simulink model "PIDcontrol"  (Simulink 8.9)
settings: Solver=ode3  StartTime=0.0  StopTime=inf  FixedStep=0.001  RelTol=1e-3  EnableMultiTasking=on
libraries: slrtlib x4, xpcquanserlib x2
settings Model: Creator=Ninad  LastModifiedBy=Rorro  SimulationMode=external
settings SolverCC: EnableConcurrentExecution=on
settings OptimizationCC: BlockReduction=off  OptimizeBlockIOStorage=off  BufferReuse=off  GlobalBufferReuse=off  ExpressionFolding=off  ExpressionDepthLimit=2147483647  LocalBlockOutputs=off
settings DebuggingCC: SolverPrmCheckMsg=warning
settings HardwareCC: ProdIntDivRoundTo=Zero  ProdEndianess=LittleEndian  ProdLongLongMode=on  ProdHWDeviceType=Generic->32-bit x86 compatible
settings RTWCC: SystemTargetFile=slrt.tlc  TemplateMakefile=slrt_default_tmf  Description=Simulink Real-Time  CodeExecutionProfiling=on  RTWCompilerOptimization=on
settings SimulinkRealTimeCC: GeneratePreprocessorConditionals=Disable all
settings ConfigComp: CovSFcnEnable=off

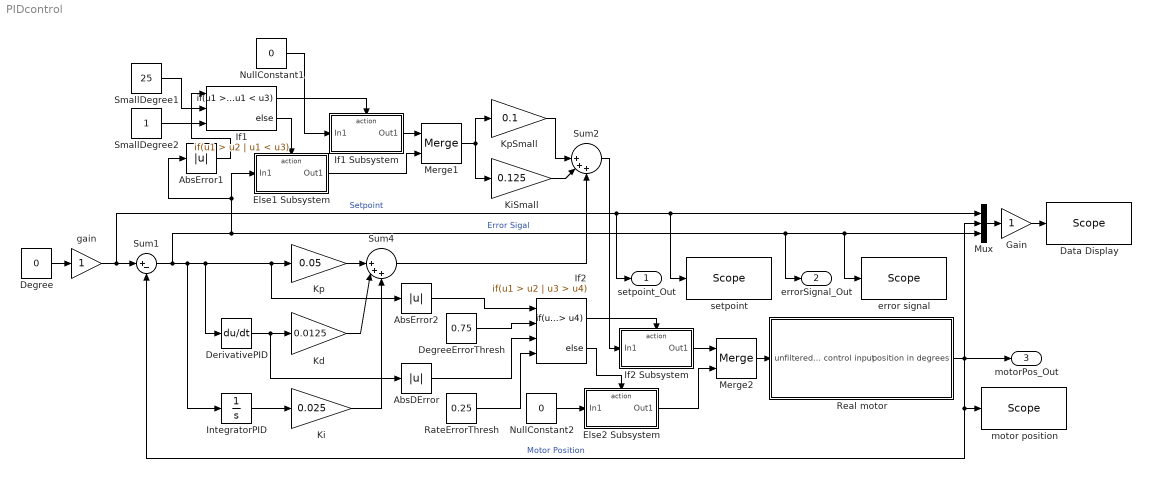
== system PIDcontrol ==
  AbsDError : Abs
  AbsError1 : Abs
  AbsError2 : Abs
  Data Display : slrtlib/Displays and Logging/Scope   scopeno=3  scopetype=Target  autostart=on  viewmode=Numerical  formatstr="'Setpoint        %3.2f,Motor Position  %3.2f,Error Signal    %3.2f'"  grid=on  ylimits=[0,170]  nosamples=200  noprepostsamples=0  interleave=10  triggermode=FreeRun  triggersignal=1  trigsignalfromport=off  triggerlevel=0.0  triggerslope=Either  triggerscope=1  triggersample=0  filename=data.dat  mode=Lazy  writesize=512  autorestart=off  dynamicfilemode=off  maxwritefilesize=512*1024^2
  Degree : Constant  Value=0
  DegreeErrorThresh : Constant  Value=0.75
  DerivativePID : Derivative
  Else1 Subsystem : Subsystem  TreatAsAtomicUnit=on
  Else2 Subsystem : Subsystem  TreatAsAtomicUnit=on
  Gain : Gain
  If1 : If  NumInputs=3  IfExpression=u1 > u2 | u1 < u3
  If1 Subsystem : Subsystem  TreatAsAtomicUnit=on
  If2 : If  NumInputs=4  IfExpression=u1 > u2 | u3 > u4
  If2 Subsystem : Subsystem  TreatAsAtomicUnit=on
  IntegratorPID : Integrator
  Kd : Gain  Gain=0.0125
  Ki : Gain  Gain=0.025
  KiSmall : Gain  Gain=0.125
  Kp : Gain  Gain=0.05
  KpSmall : Gain  Gain=0.1
  Merge1 : Merge
  Merge2 : Merge
  Mux : Mux  Inputs=3
  NullConstant1 : Constant  Value=0
  NullConstant2 : Constant  Value=0
  RateErrorThresh : Constant  Value=0.25
  Real motor : Subsystem
  SmallDegree1 : Constant  Value=25
  SmallDegree2 : Constant
  Sum1 : Sum  Inputs=|+-
  Sum2 : Sum  Inputs=||+++
  Sum4 : Sum  Inputs=||+++
  error signal : slrtlib/Displays and Logging/Scope   scopeno=2  scopetype=Target  autostart=on  viewmode=Graphical rolling  formatstr='%15.6f'  grid=on  ylimits=[-180,180]  nosamples=500  noprepostsamples=0  interleave=10  triggermode=FreeRun  triggersignal=1  trigsignalfromport=off  triggerlevel=0.0  triggerslope=Either  triggerscope=1  triggersample=0  filename=data.dat  mode=Lazy  writesize=512  autorestart=off  dynamicfilemode=off  maxwritefilesize=512*1024^2
  gain : Gain
  motor position : slrtlib/Displays and Logging/Scope   scopeno=7  scopetype=Target  autostart=on  viewmode=Graphical rolling  formatstr='%15.6f'  grid=on  ylimits=[-180,180]  nosamples=500  noprepostsamples=0  interleave=10  triggermode=FreeRun  triggersignal=1  trigsignalfromport=off  triggerlevel=0.0  triggerslope=Either  triggerscope=1  triggersample=0  filename=data.dat  mode=Lazy  writesize=512  autorestart=off  dynamicfilemode=off  maxwritefilesize=512*1024^2
  setpoint : slrtlib/Displays and Logging/Scope   scopeno=1  scopetype=Target  autostart=on  viewmode=Graphical rolling  formatstr='%15.6f'  grid=on  ylimits=[-180,180]  nosamples=500  noprepostsamples=0  interleave=10  triggermode=FreeRun  triggersignal=1  trigsignalfromport=off  triggerlevel=0.0  triggerslope=Either  triggerscope=1  triggersample=0  filename=data.dat  mode=Lazy  writesize=512  autorestart=off  dynamicfilemode=off  maxwritefilesize=512*1024^2
  setpoint_Out : Outport
  errorSignal_Out : Outport  Port=2
  motorPos_Out : Outport  Port=3
  wires:
  Kd/1 -> Sum4/2
  DerivativePID/1 -> AbsDError/1, Kd/1
  IntegratorPID/1 -> Ki/1
  Ki/1 -> Sum4/3
  gain/1 -> Sum1/1, Mux/1, setpoint/1, setpoint_Out/1  "Setpoint"
  Degree/1 -> gain/1
  Real motor/1(position in degrees) -> Sum1/2, motor position/1, motorPos_Out/1, Mux/2  "Motor Position"
  Gain/1 -> Data Display/1
  Mux/1 -> Gain/1
  Sum1/1 -> AbsError2/1, Kp/1, DerivativePID/1, IntegratorPID/1, AbsError1/1, Else1 Subsystem/1(In1), error signal/1, Mux/3, errorSignal_Out/1  "Error Sigal"
  Else2 Subsystem/1(Out1) -> Merge2/2
  If2 Subsystem/1(Out1) -> Merge2/1
  NullConstant2/1 -> Else2 Subsystem/1(In1)
  AbsError2/1 -> If2/1
  AbsDError/1 -> If2/3
  DegreeErrorThresh/1 -> If2/2
  RateErrorThresh/1 -> If2/4
  If2/1 -> If2 Subsystem/Action
  If2/2 -> Else2 Subsystem/Action
  Merge2/1 -> Real motor/1(unfiltered  control input)
  Kp/1 -> Sum4/1
  If1/1 -> If1 Subsystem/Action
  If1/2 -> Else1 Subsystem/Action
  Sum2/1 -> If2 Subsystem/1(In1)
  Sum4/1 -> Sum2/3
  KiSmall/1 -> Sum2/2
  KpSmall/1 -> Sum2/1
  If1 Subsystem/1(Out1) -> Merge1/1
  Else1 Subsystem/1(Out1) -> Merge1/2
  Merge1/1 -> KpSmall/1, KiSmall/1
  AbsError1/1 -> If1/1
  NullConstant1/1 -> If1 Subsystem/1(In1)
  SmallDegree2/1 -> If1/3
  SmallDegree1/1 -> If1/2

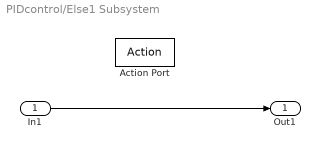
== system PIDcontrol/Else1 Subsystem ==
  In1 : Inport
  Action Port : ActionPort  ActionType=else
  Out1 : Outport
  wires:
  In1/1 -> Out1/1

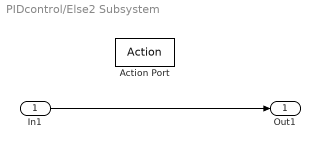
== system PIDcontrol/Else2 Subsystem ==
  In1 : Inport
  Action Port : ActionPort  ActionType=else
  Out1 : Outport
  wires:
  In1/1 -> Out1/1

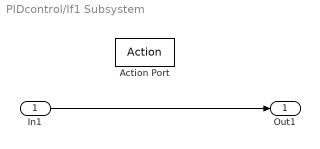
== system PIDcontrol/If1 Subsystem ==
  In1 : Inport
  Action Port : ActionPort  ActionType=then
  Out1 : Outport
  wires:
  In1/1 -> Out1/1

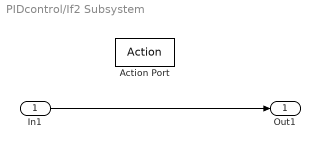
== system PIDcontrol/If2 Subsystem ==
  In1 : Inport
  Action Port : ActionPort  ActionType=then
  Out1 : Outport
  wires:
  In1/1 -> Out1/1

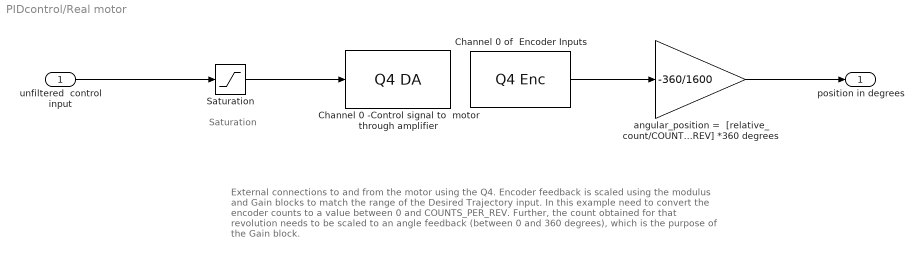
== system PIDcontrol/Real motor ==
  note: Saturation
  note: External connections to and from the motor using the Q4.
      |
      | Encoder feedback is scaled using the modulus and Gain blocks to
      | match the range of the Desired Trajectory input.
      |
      | In this example need to convert the encoder counts to a value between 0 and COUNTS_PER_REV.
      | Further, the count obtained for that revolution needs to be scaled to an angle feedback (between
      | 0 and 360 degrees), which is the purpose of the Gain block.
  unfiltered  control input : Inport
  "Channel 0 -Control signal to  motor through amplifier " : xpcquanserlib/D//A/Q4 DA   channel=[1]  range=[-10]  simul=off  reset=[1]  initValue=[0]  sampleTime=.001  slot=-1
      settings: SourceProductName=Simulink Real-Time  SourceProductBaseCode=XP
  "Channel 0 of  Encoder Inputs " : xpcquanserlib/Incremental Encoder/Q4 Enc   channel=[1]  initialCount=[0]  prescale=[1]  quadrature=[4]  mode=[0]  synchronousIndex=[0]  indexPolarity=[0]  preserveCounts=[0]  sampleTime=.001  slot=-1
      settings: SourceProductName=Simulink Real-Time  SourceProductBaseCode=XP
  Saturation : Saturate  UpperLimit=5  LowerLimit=-5
  angular_position =  [relative_count/COUNTS_PER_REV] *360 degrees : Gain  Gain=-360/1600
  position in degrees : Outport
  wires:
  Saturation/1 -> "Channel 0 -Control signal to  motor through amplifier "/1
  angular_position =  [relative_count/COUNTS_PER_REV] *360 degrees/1 -> position in degrees/1
  "Channel 0 of  Encoder Inputs "/1 -> angular_position =  [relative_count/COUNTS_PER_REV] *360 degrees/1
  unfiltered  control input/1 -> Saturation/1
